simulink subsystem "mission_file_parser"  (R2025b)
settings: Solver=VariableStepAuto  StartTime=0.0  StopTime=10.0  RelTol=1e-3
undefined symbols (not defined in the file or in its folder): dt_control, dt_data
settings Model: Creator=koryh  LastModifiedBy=kjhaydon

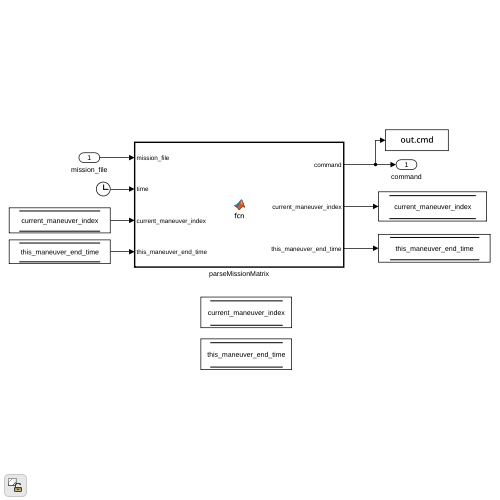
[thumbnail: Simulink's stored preview of the top-level diagram]
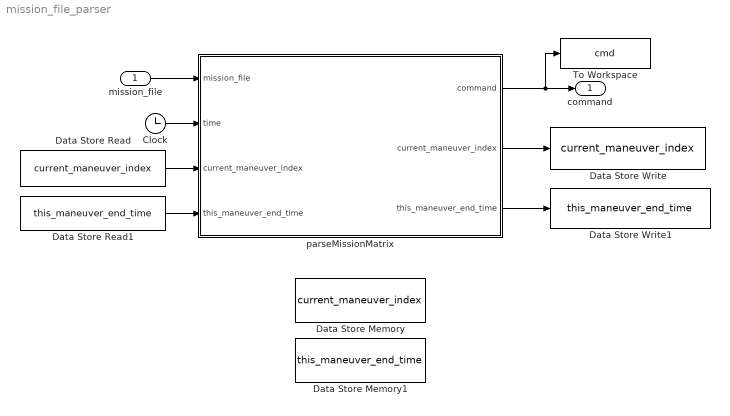
== system mission_file_parser ==
  mission_file : Inport  SampleTime=dt_control
  Clock : Clock
  Data Store Memory : DataStoreMemory  DataStoreName=current_maneuver_index  WriteAfterWriteMsg=warning  InitialValue=1  ShowAdditionalParam=off
  Data Store Memory1 : DataStoreMemory  DataStoreName=this_maneuver_end_time  WriteAfterWriteMsg=warning  InitialValue=-1  ShowAdditionalParam=off
  Data Store Read : DataStoreRead  DataStoreName=current_maneuver_index  IndexOptions=Index vector (dialog)  Indices=1  OutputSizes=1
  Data Store Read1 : DataStoreRead  DataStoreName=this_maneuver_end_time  IndexOptions=Index vector (dialog)  Indices=1  OutputSizes=1
  Data Store Write : DataStoreWrite  DataStoreName=current_maneuver_index  IndexOptions=Index vector (dialog)  Indices=1  OutputSizes=1
  Data Store Write1 : DataStoreWrite  DataStoreName=this_maneuver_end_time  IndexOptions=Index vector (dialog)  Indices=1  OutputSizes=1
  To Workspace : ToWorkspace  VariableName=cmd  SaveFormat=Timeseries  SampleTime=dt_data
  parseMissionMatrix : MATLAB Function  TreatAsAtomicUnit=on
  command : Outport
  wires:
  Data Store Read/1 -> parseMissionMatrix/3("current_maneuver_index ")
  Data Store Read1/1 -> parseMissionMatrix/4("this_maneuver_end_time ")
  mission_file/1 -> parseMissionMatrix/1(mission_file)
  parseMissionMatrix/1(command) -> command/1, To Workspace/1
  parseMissionMatrix/2(current_maneuver_index) -> Data Store Write/1
  parseMissionMatrix/3(this_maneuver_end_time) -> Data Store Write1/1
  Clock/1 -> parseMissionMatrix/2(time)

== matlab function mission_file_parser/parseMissionMatrix ==
  data: mission_file input; command output; time input; current_maneuver_index input; this_maneuver_end_time input; current_maneuver_index output; this_maneuver_end_time output
function [command, current_maneuver_index, this_maneuver_end_time] = fcn(mission_file, time, current_maneuver_index, this_maneuver_end_time)

[command, current_maneuver_index, this_maneuver_end_time] = parseMissionMatrix(mission_file,time,...
    current_maneuver_index,this_maneuver_end_time);
